simulink model "Aufgabe_10_2_1_zufuhrband"  (R2023a)
settings: Solver=ode3  StartTime=0.0  StopTime=10.0  FixedStep=0.1  RelTol=1e-3  EnableMultiTasking=on
undefined symbols (not defined in the file): sigbuilder_block
libraries: simulink x3
settings Model: Creator=Guanyu Li  LastModifiedBy=ASUS

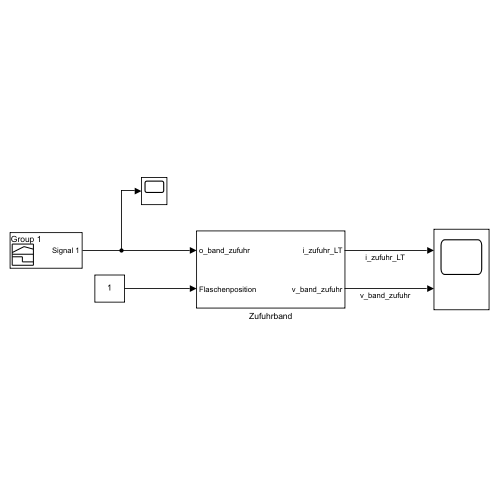
[thumbnail: Simulink's stored preview of the top-level diagram]
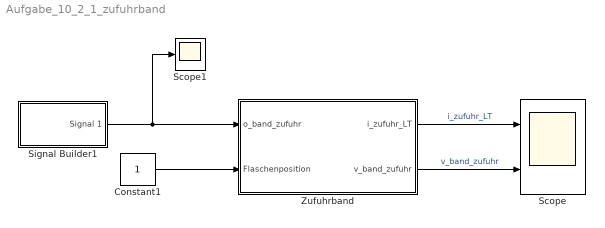
== system Aufgabe_10_2_1_zufuhrband ==
  Constant1 : Constant
  Scope : Scope  NumInputPorts=2
  Scope1 : Scope
  Signal Builder1 : Subsystem  Tag=STV Subsys  LoadFcn=sigbuilder_block('load');  StartFcn=sigbuilder_block('start');  StopFcn=sigbuilder_block('stop');  ClipboardFcn=sigbuilder_block('clipboard');  mask(Sigbuilder block){tuvar=[0:10]}
      mask help: Simulink:masks:SigbuilderBlock_MD
      mask init:
      | if ~strcmp(get_param(bdroot(gcbh),'SimulationStatus'),'stopped') tuvar = sigbuilder_block('maskInit'); end
      settings: CopyFcn=sigbuilder_block('copy');  DeleteFcn=sigbuilder_block('delete');  ModelCloseFcn=sigbuilder_block('modelClose');  PreSaveFcn=sigbuilder_block('preSave');  PauseFcn=sigbuilder_block('pause');  ContinueFcn=sigbuilder_block('continue');  NameChangeFcn=sigbuilder_block('namechange');  OpenFcn=sigbuilder_block('open',[489.5 214 551 363 ]);  CloseFcn=sigbuilder_block('close');
      mask Display: plot(0, 0, 100, 100,[2, 2, 32, 32, 2], [68, 8, 8, 68, 68],[32, 2], [38, 38], [32, 19, 2],[53, 60, 44], [32, 17, 17, 2],[16, 16, 31, 31]);txt = getActiveGroup(gcbh);text(2, 100, txt,'verticalAlignment', 'top');
  Zufuhrband : Subsystem
  wires:
  Zufuhrband/1(i_zufuhr_LT) -> Scope/1  "i_zufuhr_LT"
  Zufuhrband/2(v_band_zufuhr) -> Scope/2  "v_band_zufuhr"
  Constant1/1 -> Zufuhrband/2(Flaschenposition)
  Signal Builder1/1(Signal 1) -> Scope1/1, Zufuhrband/1(o_band_zufuhr)

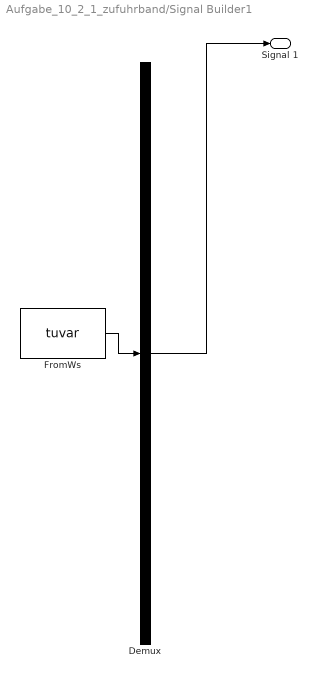
== system Aufgabe_10_2_1_zufuhrband/Signal Builder1 ==
  Demux : Demux  Tag=STV Demux  Outputs=1
      settings: DisplayOption=none
  FromWs : FromWorkspace  Tag=STV FromWs  VariableName=tuvar
      SigBuilderData=|
      | common.afterFinalStr = 'Extrapolate'
      | common.sampleTime = 0
      | dataSet.timeRange = [0 10]
      | dataSet.name = 'Group 1'
      | sbobj.Groups.Name = 'Group 1'
      | sbobj.Groups.Signals.Name = 'Signal 1'
      | sbobj.Groups.Signals.XData = [0 1 2 3 4 5 6 7 8 9 10]
      | sbobj.Groups.Signals.YData = [1 1 1 1 1 1 1 1 1 1 1]
  Signal 1 : Outport  Tag=STV Outport
  wires:
  Demux/1 -> Signal 1/1
  FromWs/1 -> Demux/1

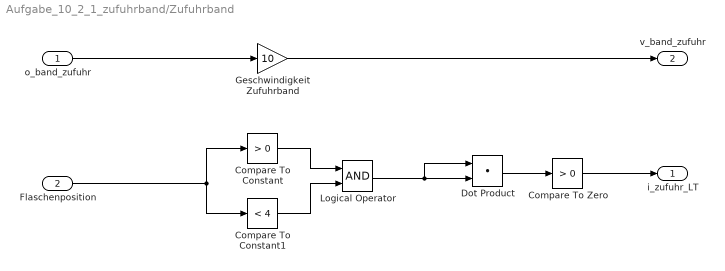
== system Aufgabe_10_2_1_zufuhrband/Zufuhrband ==
  o_band_zufuhr : Inport
  Flaschenposition : Inport  Port=2
  Compare To Constant : simulink/Logic and Bit Operations/Compare To Constant  relop=>  const=0  OutDataTypeStr=boolean
  Compare To Constant1 : simulink/Logic and Bit Operations/Compare To Constant  relop=<  const=4  OutDataTypeStr=boolean
  Compare To Zero : simulink/Logic and Bit Operations/Compare To Zero  relop=>  OutDataTypeStr=boolean
  Dot Product : DotProduct  OutDataTypeStr=Inherit: Inherit via internal rule
  Geschwindigkeit Zufuhrband : Gain  Gain=10
  Logical Operator : Logic  AllPortsSameDT=off  OutDataTypeStr=boolean
  i_zufuhr_LT : Outport
  v_band_zufuhr : Outport  Port=2
  wires:
  Compare To Constant1/1 -> Logical Operator/2
  Compare To Constant/1 -> Logical Operator/1
  o_band_zufuhr/1 -> Geschwindigkeit Zufuhrband/1
  Geschwindigkeit Zufuhrband/1 -> v_band_zufuhr/1
  Flaschenposition/1 -> Compare To Constant1/1, Compare To Constant/1
  Compare To Zero/1 -> i_zufuhr_LT/1
  Logical Operator/1 -> Dot Product/1, Dot Product/2
  Dot Product/1 -> Compare To Zero/1
